simulink model "sim_Adaptive"  (R2015a)
settings: Solver=ode4  StartTime=0.  StopTime=100  FixedStep=0.005  MaxStep=0.005  RelTol=1e-3
values from neighbouring files (symbols this model uses):
  A_ref = [0 1; -omega^2 -2*xi*omega]    [adaptive_control.m]
  B_ref = [0; omega^2]    [adaptive_control.m]
undefined symbols (not defined in the file or in its folder): C11a, G21a, M11, M21a, M21b, M22, rk, rw
settings Model: CovSFcnEnable=off  Creator=THANH DANH  LastModifiedBy=desti
settings DebuggingCC: SolverPrmCheckMsg=warning

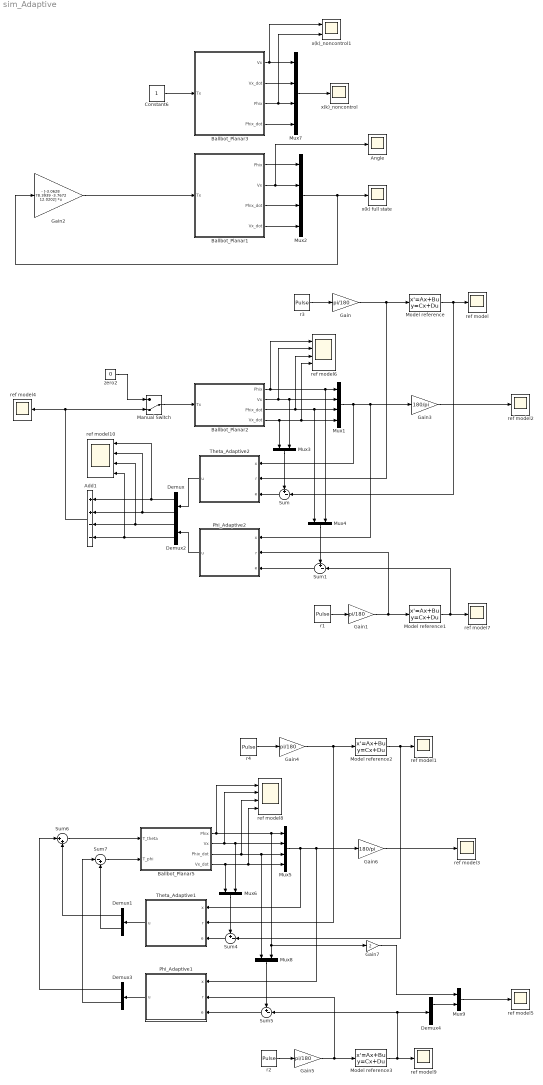
== system sim_Adaptive ==
  Add1 : Sum  Inputs=++--
  Angle : Scope
      settings: TimeRange=1  YMin=0  YMax=0.09  SaveName=Vx1
  Ballbot_Planar1 : Subsystem
  Ballbot_Planar2 : Subsystem
  Ballbot_Planar3 : Subsystem
  Ballbot_Planar5 : Subsystem
  Constant6 : Constant
  Demux{,1..4} (5 alike) : Demux  Outputs=2
  Gain{,1,4..5} (4 alike) : Gain  Gain=pi/180
  Gain2 : Gain  Gain="- [-3.0628   78.3939   -3.7672   12.0202]"  Multiplication=Matrix(K*u)
  Gain3 : Gain  Gain=180/pi
  Gain6 : Gain  Gain=180/pi
  Gain7 : Gain  Gain=2
  Manual Switch : ManualSwitch  CurrentSetting=0
  Model reference{,1..3} (4 alike) : StateSpace  A=A_ref  B=B_ref  C=[1 0; 0 1]  D=[0; 0]  X0=0
  Mux{1..2,5,7} (4 alike) : Mux
  Mux{3..4,6,8..9} (5 alike) : Mux  Inputs=2
  Phi_Adaptive1 : Subsystem
  Phi_Adaptive2 : Subsystem
  Sum{,1,4..5} (4 alike) : Sum  Inputs=+-|
  Sum6 : Sum  Inputs=|++
  Sum7 : Sum  Inputs=|-+
  Theta_Adaptive1 : Subsystem
  Theta_Adaptive2 : Subsystem
  r1 : DiscretePulseGenerator  PulseType=Time based  Amplitude=5  Period=10  PulseWidth=50  PhaseDelay=2
  r2 : DiscretePulseGenerator  PulseType=Time based  Amplitude=5  Period=10  PulseWidth=50  PhaseDelay=2
  r3 : DiscretePulseGenerator  PulseType=Time based  Amplitude=0  Period=10  PulseWidth=50  PhaseDelay=2
  r4 : DiscretePulseGenerator  PulseType=Time based  Amplitude=0  Period=10  PulseWidth=50  PhaseDelay=2
  ref model{,1..5,7,9} (8 alike) : Scope
      ref model settings: TimeRange=1  YMin=0  YMax=0.09  SaveName=Vx2
      ref model1 settings: TimeRange=1  YMin=0  YMax=0.09  SaveName=Vx3
      ref model2 settings: TimeRange=1  YMin=0  YMax=0.09  SaveName=Vx4
      ref model3 settings: TimeRange=1  YMin=0  YMax=0.09  SaveName=Vx5
      ref model4 settings: TimeRange=1  YMin=0  YMax=0.09  SaveName=Vx7
      ref model5 settings: TimeRange=1  YMin=0  YMax=0.09  SaveName=Vx8
      ref model7 settings: TimeRange=1  YMin=0  YMax=0.09  SaveName=Vx10
      ref model9 settings: TimeRange=1  YMin=0  YMax=0.09  SaveName=Vx12
  ref model10 : Scope  NumInputPorts=4
      settings: TimeRange=1  YMin=0~-5~-5~-5  YMax=0.09~5~5~5  SaveName=Vx13
  ref model6 : Scope  NumInputPorts=4
      settings: TimeRange=1  YMin=0~-5~-5~-5  YMax=0.09~5~5~5  SaveName=Vx9
  ref model8 : Scope  NumInputPorts=4
      settings: TimeRange=1  YMin=0~-5~-5~-5  YMax=0.09~5~5~5  SaveName=Vx11
  x(k) full state : Scope
      settings: TimeRange=1  YMin=0  YMax=0.09  SaveName=Vx
  x(k)_noncontrol : Scope
      settings: TimeRange=1  YMin=0  YMax=0.09  SaveName=Vx6
  x(k)_noncontrol1 : Scope  NumInputPorts=2
      settings: TimeRange=1  YMin=0~-5  YMax=0.09~5  SaveName=Vx14
  zero2 : Constant  Value=0
  wires:
  Constant6/1 -> Ballbot_Planar3/1(Tx)
  Mux7/1 -> x(k)_noncontrol/1
  Ballbot_Planar3/1(Vx) -> x(k)_noncontrol1/1, Mux7/1
  Ballbot_Planar3/2(Vx_dot) -> Mux7/2
  Ballbot_Planar3/3(Phix) -> x(k)_noncontrol1/2, Mux7/3
  Ballbot_Planar3/4(Phix_dot) -> Mux7/4
  Mux2/1 -> x(k) full state/1, Gain2/1
  Ballbot_Planar1/1(Phix) -> Mux2/1
  Ballbot_Planar1/2(Vx) -> Angle/1, Mux2/2
  Ballbot_Planar1/3(Phix_dot) -> Mux2/3
  Ballbot_Planar1/4(Vx_dot) -> Mux2/4
  Sum/1 -> Theta_Adaptive2/3(e)
  Sum1/1 -> Phi_Adaptive2/3(e)
  Mux1/1 -> Theta_Adaptive2/1(x), Phi_Adaptive2/1(x), Gain3/1
  Ballbot_Planar2/1(Phix) -> ref model6/1, Mux1/1, Mux4/2
  Ballbot_Planar2/2(Vx) -> ref model6/2, Mux1/2, Mux3/2
  Ballbot_Planar2/3(Phix_dot) -> ref model6/3, Mux1/3, Mux4/1
  Ballbot_Planar2/4(Vx_dot) -> ref model6/4, Mux1/4, Mux3/1
  Mux3/1 -> Sum/1
  Mux4/1 -> Sum1/1
  r3/1 -> Gain/1
  Model reference/1 -> ref model/1, Sum/2
  Theta_Adaptive2/1(u) -> Demux/1
  Phi_Adaptive2/1(u) -> Demux2/1
  Gain2/1 -> Ballbot_Planar1/1(Tx)
  Manual Switch/1 -> Ballbot_Planar2/1(Tx)
  zero2/1 -> Manual Switch/1
  Add1/1 -> ref model4/1, Manual Switch/2
  r1/1 -> Gain1/1
  Model reference1/1 -> Sum1/2, ref model7/1
  Gain/1 -> Theta_Adaptive2/2(r), Model reference/1
  Gain1/1 -> Phi_Adaptive2/2(r), Model reference1/1
  Gain3/1 -> ref model2/1
  Demux/1 -> Add1/1, ref model10/1
  Demux/2 -> ref model10/2, Add1/2
  Demux2/1 -> ref model10/3, Add1/3
  Demux2/2 -> ref model10/4, Add1/4
  Sum4/1 -> Theta_Adaptive1/3(e)
  Sum5/1 -> Phi_Adaptive1/3(e)
  Mux5/1 -> Gain6/1, Phi_Adaptive1/1(x), Theta_Adaptive1/1(x)
  Ballbot_Planar5/1(Phix) -> ref model8/1, Mux5/1, Gain7/1, Mux8/2
  Ballbot_Planar5/2(Vx) -> ref model8/2, Mux5/2, Mux6/2
  Ballbot_Planar5/3(Phix_dot) -> ref model8/3, Mux5/3, Mux8/1
  Ballbot_Planar5/4(Vx_dot) -> ref model8/4, Mux5/4, Mux6/1
  Mux6/1 -> Sum4/1
  Mux8/1 -> Sum5/1
  r4/1 -> Gain4/1
  Model reference2/1 -> ref model1/1, Sum4/2
  Theta_Adaptive1/1(u) -> Demux1/1
  Phi_Adaptive1/1(u) -> Demux3/1
  r2/1 -> Gain5/1
  Model reference3/1 -> Demux4/1, Sum5/2, ref model9/1
  Gain4/1 -> Model reference2/1, Theta_Adaptive1/2(r)
  Gain5/1 -> Phi_Adaptive1/2(r), Model reference3/1
  Gain6/1 -> ref model3/1
  Sum7/1 -> Ballbot_Planar5/2(T_phi)
  Sum6/1 -> Ballbot_Planar5/1(T_theta)
  Demux1/1 -> Sum6/2
  Demux3/1 -> Sum6/1
  Demux1/2 -> Sum7/2
  Demux3/2 -> Sum7/1
  Mux9/1 -> ref model5/1
  Demux4/1 -> Mux9/2
  Gain7/1 -> Mux9/1

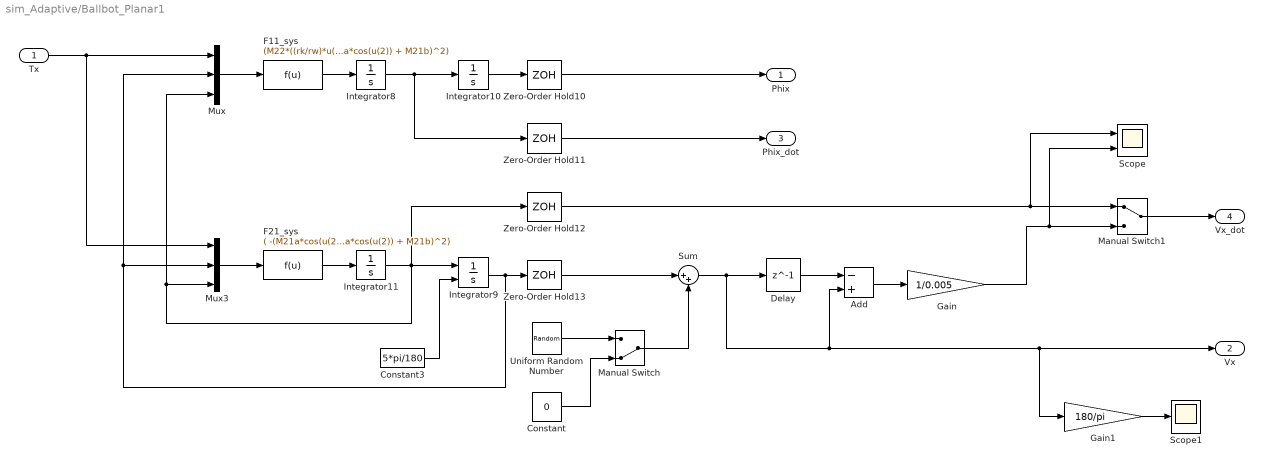
== system sim_Adaptive/Ballbot_Planar1 ==
  Tx : Inport
  Add : Sum  Inputs=-+
  Constant : Constant  Value=0
  Constant3 : Constant  Value=5*pi/180
  Delay : Delay  DelayLength=1
  F11_sys : Fcn  Expr=(M22*((rk/rw)*u(1) - C11a*sin(u(2))*(u(3))^2) - (M21a*cos(u(2)) + M21b)*((rk/rw)*u(1) - G21a*sin(u(2)))) / (M11*M22 - (M21a*cos(u(2)) + M21b)^2)
  F21_sys : Fcn  Expr=( -(M21a*cos(u(2)) + M21b)*((rk/rw)*u(1) - C11a*sin(u(2))*(u(3))^2) + M11*((rk/rw)*u(1) - G21a*sin(u(2))) ) / (M11*M22 - (M21a*cos(u(2)) + M21b)^2)
  Gain : Gain  Gain=1/0.005
  Gain1 : Gain  Gain=180/pi
  Integrator10 : Integrator
  Integrator11 : Integrator
  Integrator8 : Integrator
  Integrator9 : Integrator  InitialConditionSource=external
  Manual Switch : ManualSwitch  CurrentSetting=0
  Manual Switch1 : ManualSwitch
  Mux : Mux  Inputs=3
  Mux3 : Mux  Inputs=3
  Scope : Scope  NumInputPorts=2
      settings: YMin=-5~-5  YMax=5~5  SaveName=ScopeData6
  Scope1 : Scope
      settings: SaveName=ScopeData7
  Sum : Sum  Inputs=|++
  Uniform Random Number : UniformRandomNumber  Minimum=-0.2*pi/180  Maximum=0.2*pi/180  SampleTime=0.005
  Zero-Order Hold{10..13} (4 alike) : ZeroOrderHold  SampleTime=0.005
  Phix : Outport
  Vx : Outport  Port=2
  Phix_dot : Outport  Port=3
  Vx_dot : Outport  Port=4
  wires:
  Gain1/1 -> Scope1/1
  Manual Switch1/1 -> Vx_dot/1
  Manual Switch/1 -> Sum/2
  Constant/1 -> Manual Switch/2
  Uniform Random Number/1 -> Manual Switch/1
  Gain/1 -> Manual Switch1/2, Scope/2
  Add/1 -> Gain/1
  Delay/1 -> Add/1
  Sum/1 -> Add/2, Vx/1, Gain1/1, Delay/1
  Zero-Order Hold13/1 -> Sum/1
  Zero-Order Hold12/1 -> Manual Switch1/1, Scope/1
  Zero-Order Hold11/1 -> Phix_dot/1
  Zero-Order Hold10/1 -> Phix/1
  Constant3/1 -> Integrator9/2
  Tx/1 -> Mux/1, Mux3/1
  F11_sys/1 -> Integrator8/1
  Mux/1 -> F11_sys/1
  Mux3/1 -> F21_sys/1
  F21_sys/1 -> Integrator11/1
  Integrator9/1 -> Mux3/2, Mux/2, Zero-Order Hold13/1
  Integrator10/1 -> Zero-Order Hold10/1
  Integrator8/1 -> Zero-Order Hold11/1, Integrator10/1
  Integrator11/1 -> Mux3/3, Mux/3, Zero-Order Hold12/1, Integrator9/1

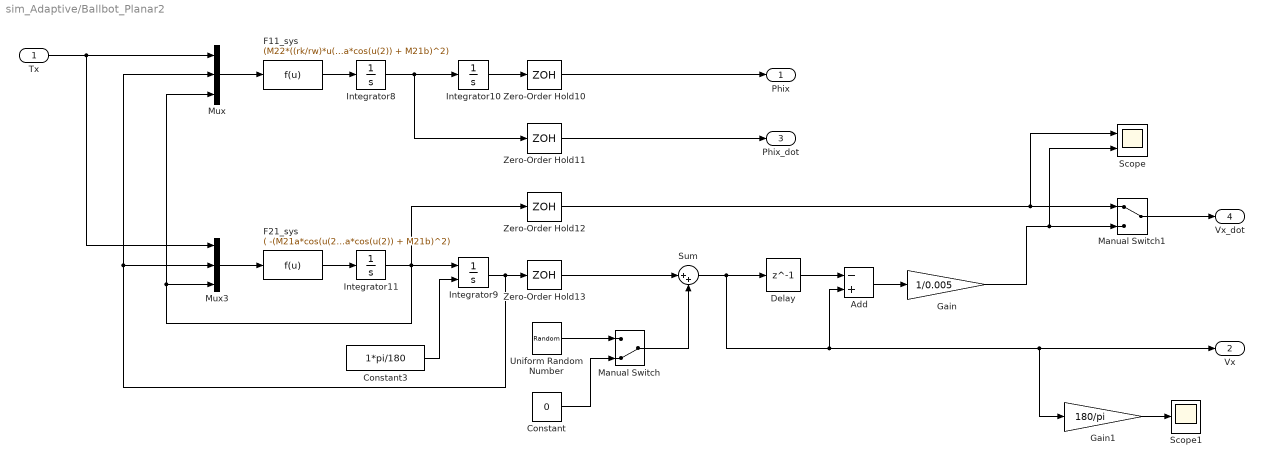
== system sim_Adaptive/Ballbot_Planar2 ==
  Tx : Inport  PortDimensions=1
  Add : Sum  Inputs=-+
  Constant : Constant  Value=0
  Constant3 : Constant  Value=1*pi/180
  Delay : Delay  DelayLength=1
  F11_sys : Fcn  Expr=(M22*((rk/rw)*u(1) - C11a*sin(u(2))*(u(3))^2) - (M21a*cos(u(2)) + M21b)*((rk/rw)*u(1) - G21a*sin(u(2)))) / (M11*M22 - (M21a*cos(u(2)) + M21b)^2)
  F21_sys : Fcn  Expr=( -(M21a*cos(u(2)) + M21b)*((rk/rw)*u(1) - C11a*sin(u(2))*(u(3))^2) + M11*((rk/rw)*u(1) - G21a*sin(u(2))) ) / (M11*M22 - (M21a*cos(u(2)) + M21b)^2)
  Gain : Gain  Gain=1/0.005
  Gain1 : Gain  Gain=180/pi
  Integrator10 : Integrator
  Integrator11 : Integrator
  Integrator8 : Integrator
  Integrator9 : Integrator  InitialConditionSource=external
  Manual Switch : ManualSwitch  CurrentSetting=0
  Manual Switch1 : ManualSwitch
  Mux : Mux  Inputs=3
  Mux3 : Mux  Inputs=3
  Scope : Scope  NumInputPorts=2
      settings: YMin=-5~-5  YMax=5~5  SaveName=ScopeData6
  Scope1 : Scope
      settings: SaveName=ScopeData7
  Sum : Sum  Inputs=|++
  Uniform Random Number : UniformRandomNumber  Minimum=-0.2*pi/180  Maximum=0.2*pi/180  SampleTime=0.005
  Zero-Order Hold{10..13} (4 alike) : ZeroOrderHold  SampleTime=0.005
  Phix : Outport  PortDimensions=1
  Vx : Outport  Port=2  PortDimensions=1
  Phix_dot : Outport  Port=3  PortDimensions=1
  Vx_dot : Outport  Port=4  PortDimensions=1
  wires:
  Integrator11/1 -> Integrator9/1, Zero-Order Hold12/1, Mux/3, Mux3/3
  Integrator8/1 -> Integrator10/1, Zero-Order Hold11/1
  Integrator10/1 -> Zero-Order Hold10/1
  Integrator9/1 -> Zero-Order Hold13/1, Mux/2, Mux3/2
  F21_sys/1 -> Integrator11/1
  Mux3/1 -> F21_sys/1
  Mux/1 -> F11_sys/1
  F11_sys/1 -> Integrator8/1
  Tx/1 -> Mux3/1, Mux/1
  Constant3/1 -> Integrator9/2
  Zero-Order Hold10/1 -> Phix/1
  Zero-Order Hold11/1 -> Phix_dot/1
  Zero-Order Hold12/1 -> Scope/1, Manual Switch1/1
  Zero-Order Hold13/1 -> Sum/1
  Sum/1 -> Delay/1, Gain1/1, Vx/1, Add/2
  Delay/1 -> Add/1
  Add/1 -> Gain/1
  Gain/1 -> Scope/2, Manual Switch1/2
  Uniform Random Number/1 -> Manual Switch/1
  Constant/1 -> Manual Switch/2
  Manual Switch/1 -> Sum/2
  Manual Switch1/1 -> Vx_dot/1
  Gain1/1 -> Scope1/1

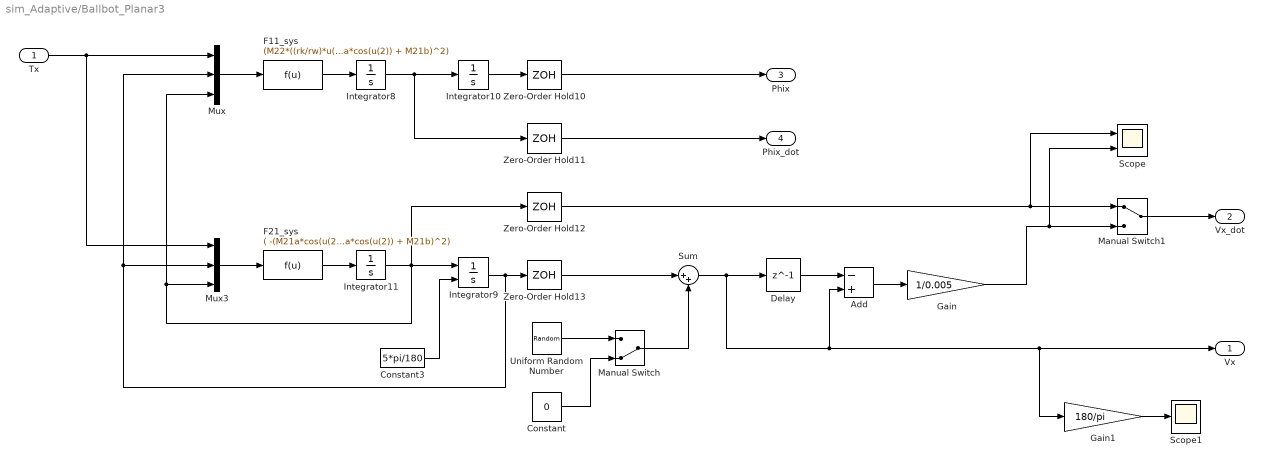
== system sim_Adaptive/Ballbot_Planar3 ==
  Tx : Inport
  Add : Sum  Inputs=-+
  Constant : Constant  Value=0
  Constant3 : Constant  Value=5*pi/180
  Delay : Delay  DelayLength=1
  F11_sys : Fcn  Expr=(M22*((rk/rw)*u(1) - C11a*sin(u(2))*(u(3))^2) - (M21a*cos(u(2)) + M21b)*((rk/rw)*u(1) - G21a*sin(u(2)))) / (M11*M22 - (M21a*cos(u(2)) + M21b)^2)
  F21_sys : Fcn  Expr=( -(M21a*cos(u(2)) + M21b)*((rk/rw)*u(1) - C11a*sin(u(2))*(u(3))^2) + M11*((rk/rw)*u(1) - G21a*sin(u(2))) ) / (M11*M22 - (M21a*cos(u(2)) + M21b)^2)
  Gain : Gain  Gain=1/0.005
  Gain1 : Gain  Gain=180/pi
  Integrator10 : Integrator
  Integrator11 : Integrator
  Integrator8 : Integrator
  Integrator9 : Integrator  InitialConditionSource=external
  Manual Switch : ManualSwitch  CurrentSetting=0
  Manual Switch1 : ManualSwitch
  Mux : Mux  Inputs=3
  Mux3 : Mux  Inputs=3
  Scope : Scope  NumInputPorts=2
      settings: YMin=-5~-5  YMax=5~5  SaveName=ScopeData6
  Scope1 : Scope
      settings: SaveName=ScopeData7
  Sum : Sum  Inputs=|++
  Uniform Random Number : UniformRandomNumber  Minimum=-0.2*pi/180  Maximum=0.2*pi/180  SampleTime=0.005
  Zero-Order Hold{10..13} (4 alike) : ZeroOrderHold  SampleTime=0.005
  Vx : Outport
  Vx_dot : Outport  Port=2
  Phix : Outport  Port=3
  Phix_dot : Outport  Port=4
  wires:
  Integrator11/1 -> Integrator9/1, Zero-Order Hold12/1, Mux/3, Mux3/3
  Integrator8/1 -> Integrator10/1, Zero-Order Hold11/1
  Integrator10/1 -> Zero-Order Hold10/1
  Integrator9/1 -> Zero-Order Hold13/1, Mux/2, Mux3/2
  F21_sys/1 -> Integrator11/1
  Mux3/1 -> F21_sys/1
  Mux/1 -> F11_sys/1
  F11_sys/1 -> Integrator8/1
  Tx/1 -> Mux3/1, Mux/1
  Constant3/1 -> Integrator9/2
  Zero-Order Hold10/1 -> Phix/1
  Zero-Order Hold11/1 -> Phix_dot/1
  Zero-Order Hold12/1 -> Scope/1, Manual Switch1/1
  Zero-Order Hold13/1 -> Sum/1
  Sum/1 -> Delay/1, Gain1/1, Vx/1, Add/2
  Delay/1 -> Add/1
  Add/1 -> Gain/1
  Gain/1 -> Scope/2, Manual Switch1/2
  Uniform Random Number/1 -> Manual Switch/1
  Constant/1 -> Manual Switch/2
  Manual Switch/1 -> Sum/2
  Manual Switch1/1 -> Vx_dot/1
  Gain1/1 -> Scope1/1

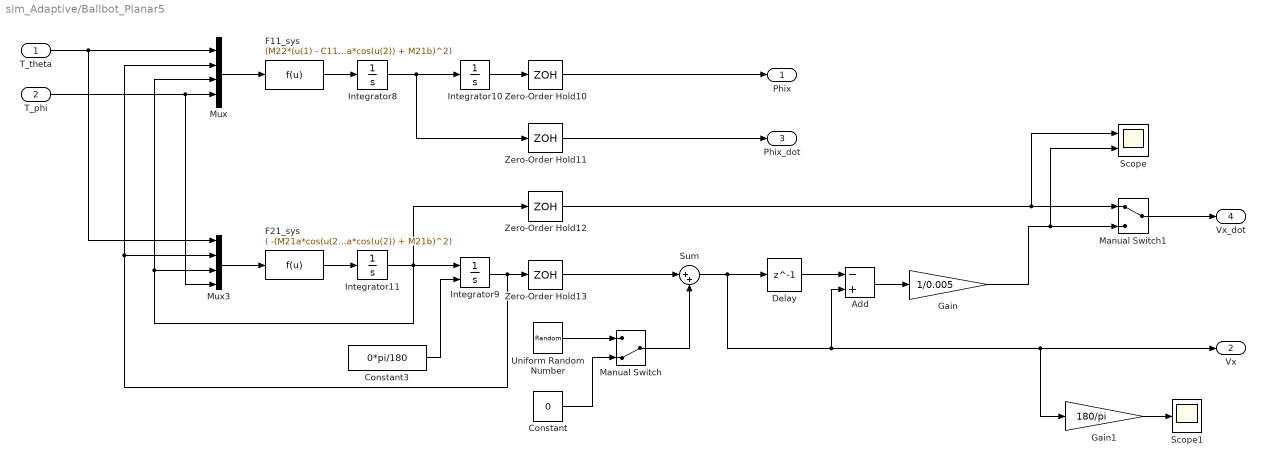
== system sim_Adaptive/Ballbot_Planar5 ==
  T_theta : Inport  PortDimensions=1
  T_phi : Inport  Port=2  PortDimensions=1
  Add : Sum  Inputs=-+
  Constant : Constant  Value=0
  Constant3 : Constant  Value=0*pi/180
  Delay : Delay  DelayLength=1
  F11_sys : Fcn  Expr=(M22*(u(1) - C11a*sin(u(2))*(u(3))^2) - (M21a*cos(u(2)) + M21b)*(u(4) - G21a*sin(u(2)))) / (M11*M22 - (M21a*cos(u(2)) + M21b)^2)
  F21_sys : Fcn  Expr=( -(M21a*cos(u(2)) + M21b)*(u(1) - C11a*sin(u(2))*(u(3))^2) + M11*(u(4) - G21a*sin(u(2))) ) / (M11*M22 - (M21a*cos(u(2)) + M21b)^2)
  Gain : Gain  Gain=1/0.005
  Gain1 : Gain  Gain=180/pi
  Integrator10 : Integrator
  Integrator11 : Integrator
  Integrator8 : Integrator
  Integrator9 : Integrator  InitialConditionSource=external
  Manual Switch : ManualSwitch  CurrentSetting=0
  Manual Switch1 : ManualSwitch
  Mux : Mux
  Mux3 : Mux
  Scope : Scope  NumInputPorts=2
      settings: YMin=-5~-5  YMax=5~5  SaveName=ScopeData6
  Scope1 : Scope
      settings: SaveName=ScopeData7
  Sum : Sum  Inputs=|++
  Uniform Random Number : UniformRandomNumber  Minimum=-0.2*pi/180  Maximum=0.2*pi/180  SampleTime=0.005
  Zero-Order Hold{10..13} (4 alike) : ZeroOrderHold  SampleTime=0.005
  Phix : Outport  PortDimensions=1
  Vx : Outport  Port=2  PortDimensions=1
  Phix_dot : Outport  Port=3  PortDimensions=1
  Vx_dot : Outport  Port=4  PortDimensions=1
  wires:
  T_phi/1 -> Mux/4, Mux3/4
  Integrator11/1 -> Integrator9/1, Zero-Order Hold12/1, Mux/3, Mux3/3
  Integrator8/1 -> Integrator10/1, Zero-Order Hold11/1
  Integrator10/1 -> Zero-Order Hold10/1
  Integrator9/1 -> Zero-Order Hold13/1, Mux/2, Mux3/2
  F21_sys/1 -> Integrator11/1
  Mux3/1 -> F21_sys/1
  Mux/1 -> F11_sys/1
  F11_sys/1 -> Integrator8/1
  T_theta/1 -> Mux/1, Mux3/1
  Constant3/1 -> Integrator9/2
  Zero-Order Hold11/1 -> Phix_dot/1
  Zero-Order Hold12/1 -> Scope/1, Manual Switch1/1
  Zero-Order Hold13/1 -> Sum/1
  Sum/1 -> Delay/1, Gain1/1, Vx/1, Add/2
  Delay/1 -> Add/1
  Add/1 -> Gain/1
  Gain/1 -> Scope/2, Manual Switch1/2
  Uniform Random Number/1 -> Manual Switch/1
  Constant/1 -> Manual Switch/2
  Manual Switch/1 -> Sum/2
  Manual Switch1/1 -> Vx_dot/1
  Gain1/1 -> Scope1/1
  Zero-Order Hold10/1 -> Phix/1

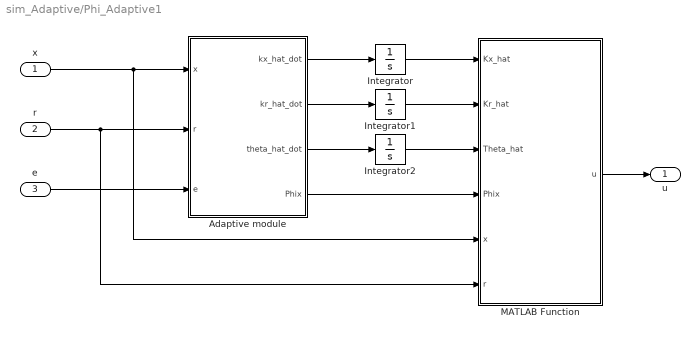
== system sim_Adaptive/Phi_Adaptive1 ==
  x : Inport  PortDimensions=4
  r : Inport  Port=2
  e : Inport  Port=3  PortDimensions=2
  Adaptive module : MATLAB Function  TreatAsAtomicUnit=on
  Integrator : Integrator  InitialCondition=1
  Integrator1 : Integrator  InitialCondition=-1
  Integrator2 : Integrator
  MATLAB Function : MATLAB Function  TreatAsAtomicUnit=on
  u : Outport  PortDimensions=2
  wires:
  Adaptive module/1(kx_hat_dot) -> Integrator/1
  Adaptive module/3(theta_hat_dot) -> Integrator2/1
  Adaptive module/2(kr_hat_dot) -> Integrator1/1
  e/1 -> Adaptive module/3(e)
  x/1 -> MATLAB Function/5(x), Adaptive module/1(x)
  r/1 -> MATLAB Function/6(r), Adaptive module/2(r)
  Integrator/1 -> MATLAB Function/1(Kx_hat)
  Integrator2/1 -> MATLAB Function/3(Theta_hat)
  Integrator1/1 -> MATLAB Function/2(Kr_hat)
  Adaptive module/4(Phix) -> MATLAB Function/4(Phix)
  MATLAB Function/1(u) -> u/1

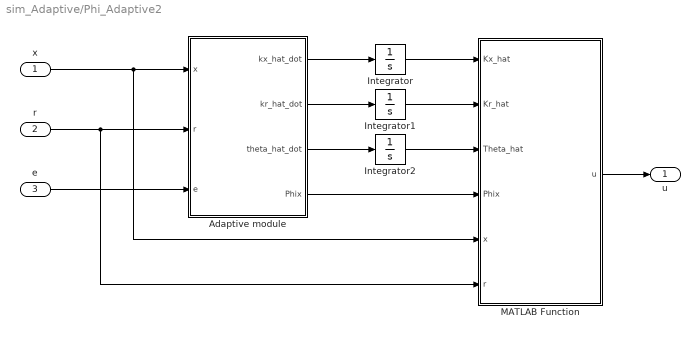
== system sim_Adaptive/Phi_Adaptive2 ==
  x : Inport  PortDimensions=4
  r : Inport  Port=2
  e : Inport  Port=3  PortDimensions=2
  Adaptive module : MATLAB Function  TreatAsAtomicUnit=on
  Integrator : Integrator  InitialCondition=1
  Integrator1 : Integrator  InitialCondition=-1
  Integrator2 : Integrator
  MATLAB Function : MATLAB Function  TreatAsAtomicUnit=on
  u : Outport  PortDimensions=2
  wires:
  MATLAB Function/1(u) -> u/1
  Adaptive module/4(Phix) -> MATLAB Function/4(Phix)
  Integrator1/1 -> MATLAB Function/2(Kr_hat)
  Integrator2/1 -> MATLAB Function/3(Theta_hat)
  Integrator/1 -> MATLAB Function/1(Kx_hat)
  r/1 -> Adaptive module/2(r), MATLAB Function/6(r)
  x/1 -> Adaptive module/1(x), MATLAB Function/5(x)
  e/1 -> Adaptive module/3(e)
  Adaptive module/2(kr_hat_dot) -> Integrator1/1
  Adaptive module/3(theta_hat_dot) -> Integrator2/1
  Adaptive module/1(kx_hat_dot) -> Integrator/1

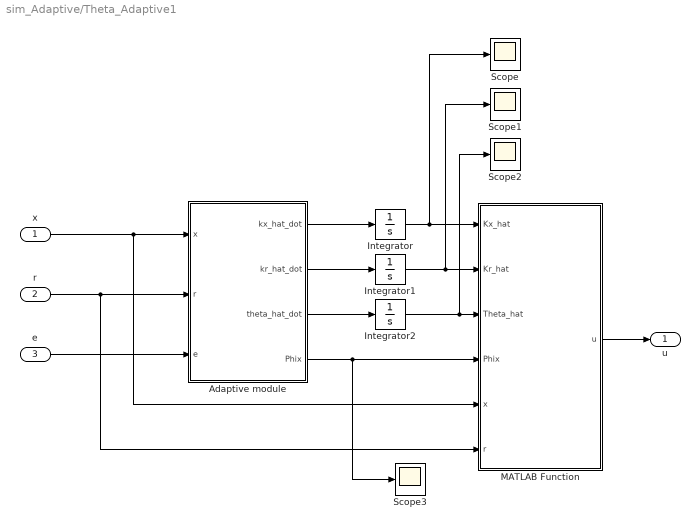
== system sim_Adaptive/Theta_Adaptive1 ==
  x : Inport  PortDimensions=4
  r : Inport  Port=2  PortDimensions=1
  e : Inport  Port=3  PortDimensions=2
  Adaptive module : MATLAB Function  TreatAsAtomicUnit=on
  Integrator : Integrator  InitialCondition=1
  Integrator1 : Integrator  InitialCondition=-1
  Integrator2 : Integrator
  MATLAB Function : MATLAB Function  TreatAsAtomicUnit=on
  Scope{,1..3} (4 alike) : Scope
      Scope2 settings: SaveName=ScopeData2
      Scope3 settings: SaveName=ScopeData3
  u : Outport  PortDimensions=2
  wires:
  Adaptive module/1(kx_hat_dot) -> Integrator/1
  Adaptive module/3(theta_hat_dot) -> Integrator2/1
  Adaptive module/2(kr_hat_dot) -> Integrator1/1
  e/1 -> Adaptive module/3(e)
  x/1 -> MATLAB Function/5(x), Adaptive module/1(x)
  r/1 -> MATLAB Function/6(r), Adaptive module/2(r)
  Integrator/1 -> Scope/1, MATLAB Function/1(Kx_hat)
  Integrator2/1 -> Scope2/1, MATLAB Function/3(Theta_hat)
  Integrator1/1 -> Scope1/1, MATLAB Function/2(Kr_hat)
  Adaptive module/4(Phix) -> Scope3/1, MATLAB Function/4(Phix)
  MATLAB Function/1(u) -> u/1

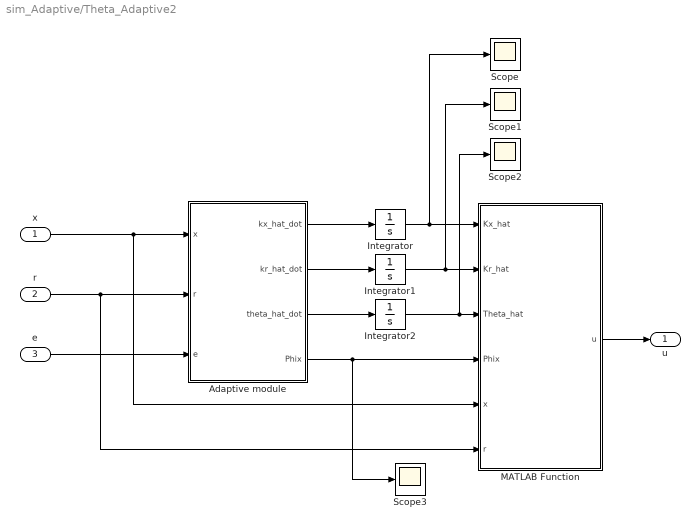
== system sim_Adaptive/Theta_Adaptive2 ==
  x : Inport  PortDimensions=4
  r : Inport  Port=2  PortDimensions=1
  e : Inport  Port=3  PortDimensions=2
  Adaptive module : MATLAB Function  TreatAsAtomicUnit=on
  Integrator : Integrator  InitialCondition=1
  Integrator1 : Integrator  InitialCondition=-1
  Integrator2 : Integrator
  MATLAB Function : MATLAB Function  TreatAsAtomicUnit=on
  Scope{,1..3} (4 alike) : Scope
      Scope2 settings: SaveName=ScopeData2
      Scope3 settings: SaveName=ScopeData3
  u : Outport  PortDimensions=2
  wires:
  MATLAB Function/1(u) -> u/1
  Adaptive module/4(Phix) -> MATLAB Function/4(Phix), Scope3/1
  Integrator1/1 -> MATLAB Function/2(Kr_hat), Scope1/1
  Integrator2/1 -> MATLAB Function/3(Theta_hat), Scope2/1
  Integrator/1 -> MATLAB Function/1(Kx_hat), Scope/1
  r/1 -> Adaptive module/2(r), MATLAB Function/6(r)
  x/1 -> Adaptive module/1(x), MATLAB Function/5(x)
  e/1 -> Adaptive module/3(e)
  Adaptive module/2(kr_hat_dot) -> Integrator1/1
  Adaptive module/3(theta_hat_dot) -> Integrator2/1
  Adaptive module/1(kx_hat_dot) -> Integrator/1

== matlab function sim_Adaptive/Phi_Adaptive1/Adaptive module ==
  data: x input; kx_hat_dot output; r input; kr_hat_dot output; theta_hat_dot output; e input; Phix output
function [kx_hat_dot,kr_hat_dot,theta_hat_dot, Phix] = fcn(x, r, e)
% % Adaptive parameters
Gama_x = [100 0; 0 300];
Gama_r = 200;
Gama_theta = diag([100 100 100]);

Phix = [x(3,:); x(2,:); x(4,:)];

%Phix = [x(3,:); 1; x(4,:)];

P = [630.2996  1.5335; 1.5335 18.9559];
B = [0 0; 1 -1];

x2 = [x(1,:); x(3,:)];

kx_hat_dot = -Gama_x*x2*e'*P*B;
kr_hat_dot = -Gama_r*r*e'*P*B;
theta_hat_dot = Gama_theta*Phix*e'*P*B;

== matlab function sim_Adaptive/Phi_Adaptive1/MATLAB Function ==
  data: u output; Kx_hat input; Kr_hat input; Theta_hat input; Phix input; x input; r input
function u = fcn(Kx_hat, Kr_hat, Theta_hat, Phix, x, r)
  
x2 = [x(1,:); x(3,:)];
u_temp = Kx_hat'*x2 + Kr_hat'*r - Theta_hat'*Phix;

u = u_temp';

== matlab function sim_Adaptive/Theta_Adaptive1/Adaptive module ==
  data: x input; kx_hat_dot output; r input; kr_hat_dot output; theta_hat_dot output; e input; Phix output
function [kx_hat_dot,kr_hat_dot,theta_hat_dot, Phix] = fcn(x, r, e)
% % Adaptive parameters
Gama_x = [9000 0; 0 3];
Gama_r = 5;
Gama_theta = diag([0.1 0.1 0.1]);


Phix = [x(3,:); x(2,:); x(4,:)];



P = [630.2996  1.5335; 1.5335 18.9559];
B = [0 0; -1 1];


x1 = [x(2,:); x(4,:)]; 

kx_hat_dot = -Gama_x*x1*e'*P*B;
kr_hat_dot = -Gama_r*r*e'*P*B;
theta_hat_dot = Gama_theta*Phix*e'*P*B;

== matlab function sim_Adaptive/Theta_Adaptive1/MATLAB Function ==
  data: u output; Kx_hat input; Kr_hat input; Theta_hat input; Phix input; x input; r input
function u = fcn(Kx_hat, Kr_hat, Theta_hat, Phix, x, r)

x1 = [x(2,:); x(4,:)];

u_temp = Kx_hat'*x1 + Kr_hat'*r - Theta_hat'*Phix;

u = u_temp';

== matlab function sim_Adaptive/Theta_Adaptive2/Adaptive module ==
  data: x input; kx_hat_dot output; r input; kr_hat_dot output; theta_hat_dot output; e input; Phix output
function [kx_hat_dot,kr_hat_dot,theta_hat_dot, Phix] = fcn(x, r, e)
% % Adaptive parameters
Gama_x = [9000 0; 0 3];
Gama_r = 5;
Gama_theta = diag([0.1 0.1 0.1]);


Phix = [x(3,:); x(2,:); x(4,:)];



P = [630.2996  1.5335; 1.5335 18.9559];
B = [0 0; -1 1];


x1 = [x(2,:); x(4,:)]; 

kx_hat_dot = -Gama_x*x1*e'*P*B;
kr_hat_dot = -Gama_r*r*e'*P*B;
theta_hat_dot = Gama_theta*Phix*e'*P*B;

== matlab function sim_Adaptive/Theta_Adaptive2/MATLAB Function ==
  data: u output; Kx_hat input; Kr_hat input; Theta_hat input; Phix input; x input; r input
function u = fcn(Kx_hat, Kr_hat, Theta_hat, Phix, x, r)

x1 = [x(2,:); x(4,:)];

u_temp = Kx_hat'*x1 + Kr_hat'*r - Theta_hat'*Phix;

u = u_temp;

== matlab function sim_Adaptive/Phi_Adaptive2/Adaptive module ==
  data: x input; kx_hat_dot output; r input; kr_hat_dot output; theta_hat_dot output; e input; Phix output
function [kx_hat_dot,kr_hat_dot,theta_hat_dot, Phix] = fcn(x, r, e)
% % Adaptive parameters
Gama_x = [100 0; 0 300];
Gama_r = 200;
Gama_theta = diag([100 100 100]);

Phix = [x(3,:); x(2,:); x(4,:)];

%Phix = [x(3,:); 1; x(4,:)];

P = [630.2996  1.5335; 1.5335 18.9559];
B = [0 0; 1 -1];

x2 = [x(1,:); x(3,:)];

kx_hat_dot = -Gama_x*x2*e'*P*B;
kr_hat_dot = -Gama_r*r*e'*P*B;
theta_hat_dot = Gama_theta*Phix*e'*P*B;

== matlab function sim_Adaptive/Phi_Adaptive2/MATLAB Function ==
  data: u output; Kx_hat input; Kr_hat input; Theta_hat input; Phix input; x input; r input
function u = fcn(Kx_hat, Kr_hat, Theta_hat, Phix, x, r)
  
x2 = [x(1,:); x(3,:)];
u_temp = Kx_hat'*x2 + Kr_hat'*r - Theta_hat'*Phix;

u = u_temp';
